simulink model "DataReceive"  (R2014a)
settings: Solver=FixedStepDiscrete  StartTime=0.0  StopTime=inf  FixedStep=0.01  RelTol=1e-3
libraries: etargetslib x1, dspnetwork x1
settings Model: Creator=ses  LastModifiedBy=ses
settings RTWCC: GenCodeOnly=on  GenerateReport=on  LaunchReport=on

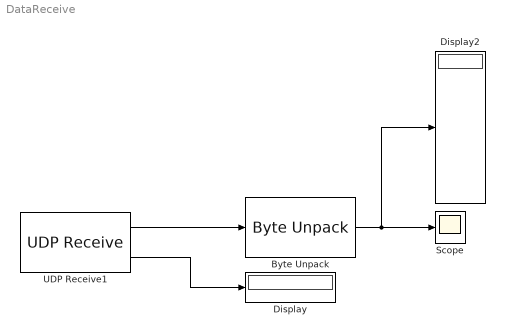
== system DataReceive ==
  Byte Unpack : etargetslib/Byte Unpack  dimensions={1}  datatypes={'double'}  byteAlign=1
  Display : Display
  Display2 : Display
  Scope : Scope
      settings: TimeRange=50
  UDP Receive1 : dspnetwork/UDP Receive  localURL='0.0.0.0'  localPort=5000  remoteURL='192.168.0.11'  remotePort=-1  recvBufferSize=512  dims=8  signalDatatype=uint8  isVarSize=off  showBlockingTime=on  blockingTime=1  sampletime=0.01  blockPlatform=WINDOWS
  wires:
  UDP Receive1/1 -> Byte Unpack/1
  Byte Unpack/1 -> Display2/1, Scope/1
  UDP Receive1/2 -> Display/1
